simulink model "rotor_simulink"  (R2022a)
settings: Solver=FixedStepAuto  StartTime=0  StopTime=150  FixedStep=time_step  RelTol=1e-3
undefined symbols (not defined in the file or in its folder): blade, gearbox, generator, I_eq, K_opt, lambda_vector, lookup_cP, omega_r, omega_rated, pitch_range, pitch_vector, rho, rotor, wind_speed
settings Model: Creator=Niccolò  LastModifiedBy=Niccolò

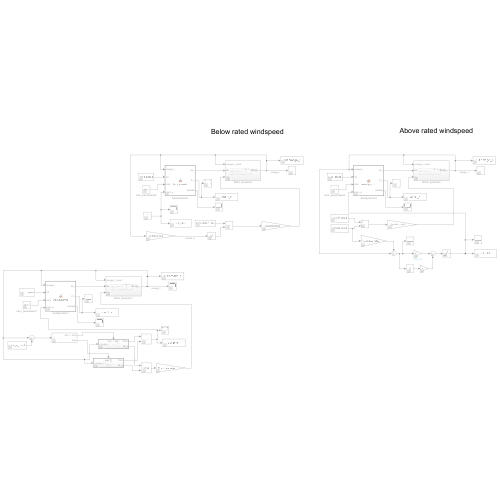
[thumbnail: Simulink's stored preview of the top-level diagram]
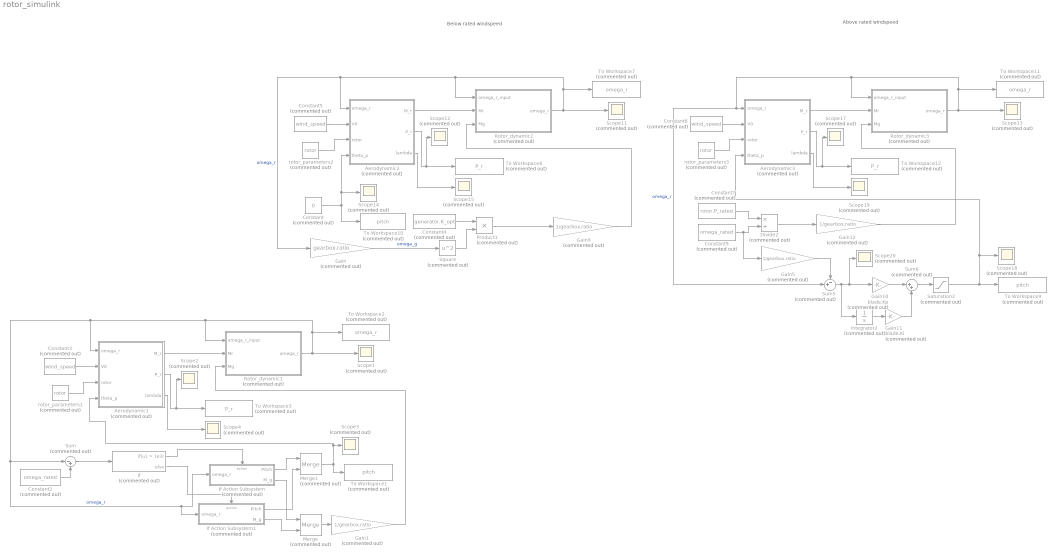
== system rotor_simulink ==
  note: Below rated windspeed
  note: Above rated windspeed
  Aerodynamic1 : MATLAB Function  Commented=on  TreatAsAtomicUnit=on
  Aerodynamic2 : MATLAB Function  Commented=on  TreatAsAtomicUnit=on
  Aerodynamic3 : MATLAB Function  Commented=on  TreatAsAtomicUnit=on
  Constant : Constant  Commented=on  Value=0
  Constant2 : Constant  Commented=on  Value=omega_rated
  Constant3 : Constant  Commented=on  Value=wind_speed
  Constant4 : Constant  Commented=on  Value=generator.K_opt
  Constant5 : Constant  Commented=on  Value=wind_speed
  Constant7 : Constant  Commented=on  Value=rotor.P_rated
  Constant8 : Constant  Commented=on  Value=wind_speed
  Constant9 : Constant  Commented=on  Value=omega_rated
  Divide2 : Product  Commented=on  Inputs=*/
  Gain : Gain  Commented=on  Gain=gearbox.ratio
  Gain{1,5,9,12} (4 alike) : Gain  Commented=on  Gain=1/gearbox.ratio
  Gain10 : Gain  Commented=on  Gain=blade.Kp
  Gain11 : Gain  Commented=on  Gain=blade.Ki
  If : If  Commented=on  IfExpression=u1 > 1e3
  If Action Subsystem : Subsystem  Commented=on  TreatAsAtomicUnit=on
  If Action Subsystem1 : Subsystem  Commented=on  TreatAsAtomicUnit=on
  Integrator2 : Integrator  Commented=on
  Merge : Merge  Commented=on
  Merge1 : Merge  Commented=on
  Product1 : Product  Commented=on
  Rotor_dynamic1 : Subsystem  Commented=on
  Rotor_dynamic2 : Subsystem  Commented=on
  Rotor_dynamic3 : Subsystem  Commented=on
  Saturation2 : Saturate  Commented=on  UpperLimit=30*pi/180  LowerLimit=pitch_range(1)
  Scope{1..4,11..15,17..20} (13 alike) : Scope  Commented=on
  Square : Math  Commented=on  Operator=square
  Sum : Sum  Commented=on  Inputs=|-+
  Sum5 : Sum  Commented=on  Inputs=-+|
  Sum6 : Sum  Commented=on  Inputs=|++
  To Workspace1 : ToWorkspace  Commented=on  VariableName=pitch  SaveFormat=Timeseries  SampleTime=-1
  To Workspace10 : ToWorkspace  Commented=on  VariableName=pitch  SaveFormat=Timeseries  SampleTime=-1
  To Workspace11 : ToWorkspace  Commented=on  VariableName=omega_r  SaveFormat=Timeseries  SampleTime=-1
  To Workspace12 : ToWorkspace  Commented=on  VariableName=P_r  SaveFormat=Timeseries  SampleTime=-1
  To Workspace2 : ToWorkspace  Commented=on  VariableName=omega_r  SaveFormat=Timeseries  SampleTime=-1
  To Workspace3 : ToWorkspace  Commented=on  VariableName=P_r  SaveFormat=Timeseries  SampleTime=-1
  To Workspace7 : ToWorkspace  Commented=on  VariableName=omega_r  SaveFormat=Timeseries  SampleTime=-1
  To Workspace8 : ToWorkspace  Commented=on  VariableName=P_r  SaveFormat=Timeseries  SampleTime=-1
  To Workspace9 : ToWorkspace  Commented=on  VariableName=pitch  SaveFormat=Timeseries  SampleTime=-1
  rotor_parameters1 : Constant  Commented=on  Value=rotor  OutDataTypeStr=Bus: rotor_bus
  rotor_parameters2 : Constant  Commented=on  Value=rotor  OutDataTypeStr=Bus: rotor_bus
  rotor_parameters3 : Constant  Commented=on  Value=rotor  OutDataTypeStr=Bus: rotor_bus
  wires:
  Rotor_dynamic2/1(omega_r) -> Scope11/1, To Workspace7/1, Rotor_dynamic2/1(omega_r_input), Gain/1, Aerodynamic2/1(omega_r)  "omega_r"
  Constant5/1 -> Aerodynamic2/2(V0)
  Aerodynamic2/2(P_r) -> Scope12/1, To Workspace8/1
  Gain9/1 -> Rotor_dynamic2/3(Mg)
  Aerodynamic2/3(lambda) -> Scope15/1
  Aerodynamic2/1(M_r) -> Rotor_dynamic2/2(Mr)
  rotor_parameters2/1 -> Aerodynamic2/3(rotor)
  Saturation2/1 -> To Workspace9/1, Scope18/1, Aerodynamic3/4(theta_p)
  Sum6/1 -> Saturation2/1
  Constant7/1 -> Divide2/1
  Gain5/1 -> Sum5/1
  rotor_parameters3/1 -> Aerodynamic3/3(rotor)
  Integrator2/1 -> Gain11/1
  Aerodynamic3/1(M_r) -> Rotor_dynamic3/2(Mr)
  Aerodynamic3/3(lambda) -> Scope19/1
  Aerodynamic3/2(P_r) -> Scope17/1, To Workspace12/1
  Divide2/1 -> Gain12/1
  Gain10/1 -> Sum6/1
  Gain12/1 -> Rotor_dynamic3/3(Mg)
  Constant8/1 -> Aerodynamic3/2(V0)
  Constant9/1 -> Gain5/1, Divide2/2
  Sum5/1 -> Scope20/1, Gain10/1, Integrator2/1
  Gain11/1 -> Sum6/2
  Rotor_dynamic3/1(omega_r) -> Scope13/1, To Workspace11/1, Rotor_dynamic3/1(omega_r_input), Sum5/2, Aerodynamic3/1(omega_r)  "omega_r"
  Constant/1 -> Aerodynamic2/4(theta_p), Scope14/1, To Workspace10/1
  Constant4/1 -> Product1/1
  Gain/1 -> Square/1  "omega_g"
  Square/1 -> Product1/2
  Product1/1 -> Gain9/1
  Aerodynamic1/2(P_r) -> Scope2/1, To Workspace3/1
  If/1 -> If Action Subsystem/Action
  If/2 -> If Action Subsystem1/Action
  Constant3/1 -> Aerodynamic1/2(V0)
  Aerodynamic1/3(lambda) -> Scope4/1
  rotor_parameters1/1 -> Aerodynamic1/3(rotor)
  Aerodynamic1/1(M_r) -> Rotor_dynamic1/2(Mr)
  Gain1/1 -> Rotor_dynamic1/3(Mg)
  Rotor_dynamic1/1(omega_r) -> Scope1/1, To Workspace2/1, Rotor_dynamic1/1(omega_r_input), Sum/1, If Action Subsystem1/1(omega_r), If Action Subsystem/1(omega_r), Aerodynamic1/1(omega_r)  "omega_r"
  If Action Subsystem/2(M_g) -> Merge/1
  If Action Subsystem1/2(M_g) -> Merge/2
  Merge/1 -> Gain1/1
  Sum/1 -> If/1
  Constant2/1 -> Sum/2
  If Action Subsystem/1(Pitch) -> Merge1/1
  If Action Subsystem1/1(Pitch) -> Merge1/2
  Merge1/1 -> To Workspace1/1, Scope3/1, Aerodynamic1/4(theta_p)

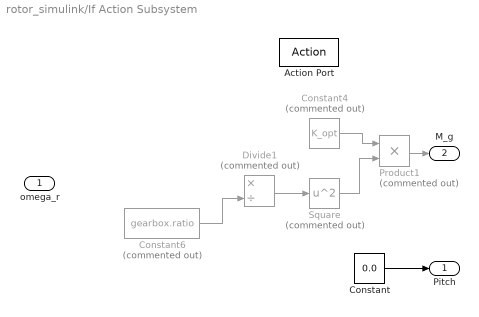
== system rotor_simulink/If Action Subsystem ==
  omega_r : Inport
  Action Port : ActionPort  ActionPortLabel=if(u1 > 1e3)
  Constant : Constant  Value=0.0
  Constant4 : Constant  Commented=on  Value=K_opt
  Constant6 : Constant  Commented=on  Value=gearbox.ratio
  Divide1 : Product  Commented=on  Inputs=*/
  Product1 : Product  Commented=on
  Square : Math  Commented=on  Operator=square
  Pitch : Outport
  M_g : Outport  Port=2
  wires:
  Square/1 -> Product1/2
  Divide1/1 -> Square/1
  Constant4/1 -> Product1/1
  Constant6/1 -> Divide1/2
  Product1/1 -> M_g/1
  Constant/1 -> Pitch/1

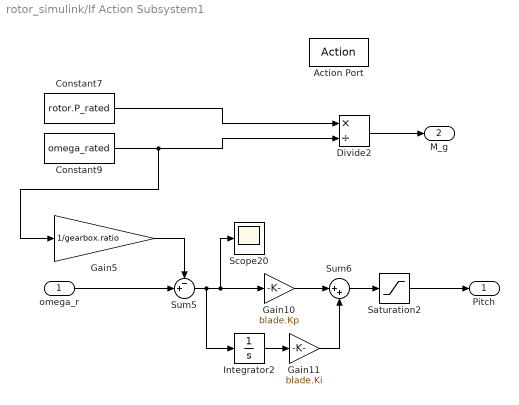
== system rotor_simulink/If Action Subsystem1 ==
  omega_r : Inport
  Action Port : ActionPort  ActionPortLabel=else
  Constant7 : Constant  Value=rotor.P_rated
  Constant9 : Constant  Value=omega_rated
  Divide2 : Product  Inputs=*/
  Gain10 : Gain  Gain=blade.Kp
  Gain11 : Gain  Gain=blade.Ki
  Gain5 : Gain  Gain=1/gearbox.ratio
  Integrator2 : Integrator
  Saturation2 : Saturate  UpperLimit=30*pi/180  LowerLimit=pitch_range(1)
  Scope20 : Scope
  Sum5 : Sum  Inputs=-+|
  Sum6 : Sum  Inputs=|++
  Pitch : Outport
  M_g : Outport  Port=2
  wires:
  Constant7/1 -> Divide2/1
  Divide2/1 -> M_g/1
  Sum6/1 -> Saturation2/1
  Integrator2/1 -> Gain11/1
  Constant9/1 -> Gain5/1, Divide2/2
  Gain11/1 -> Sum6/2
  Sum5/1 -> Scope20/1, Gain10/1, Integrator2/1
  Gain5/1 -> Sum5/1
  Gain10/1 -> Sum6/1
  Saturation2/1 -> Pitch/1
  omega_r/1 -> Sum5/2

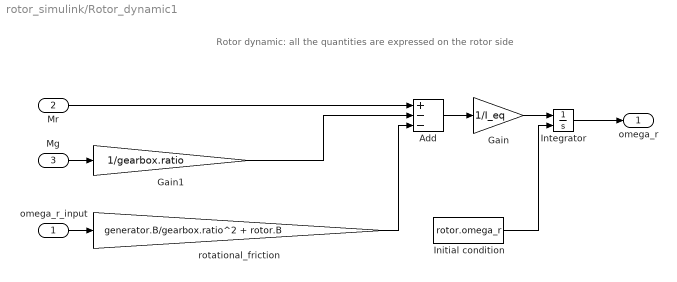
== system rotor_simulink/Rotor_dynamic1 ==
  note: Rotor dynamic: all the quantities are expressed on the rotor side
  omega_r_input : Inport
  Mr : Inport  Port=2
  Mg : Inport  Port=3
  Add : Sum  Inputs=+--
  Gain : Gain  Gain=1/I_eq
  Gain1 : Gain  Gain=1/gearbox.ratio
  Initial condition : Constant  Value=rotor.omega_r
  Integrator : Integrator  InitialConditionSource=external  InitialCondition=omega_r
  rotational_friction : Gain  Gain=generator.B/gearbox.ratio^2 + rotor.B
  omega_r : Outport
  wires:
  Add/1 -> Gain/1
  Gain/1 -> Integrator/1
  Mr/1 -> Add/1
  Initial condition/1 -> Integrator/2
  omega_r_input/1 -> rotational_friction/1
  rotational_friction/1 -> Add/3
  Mg/1 -> Gain1/1
  Gain1/1 -> Add/2
  Integrator/1 -> omega_r/1

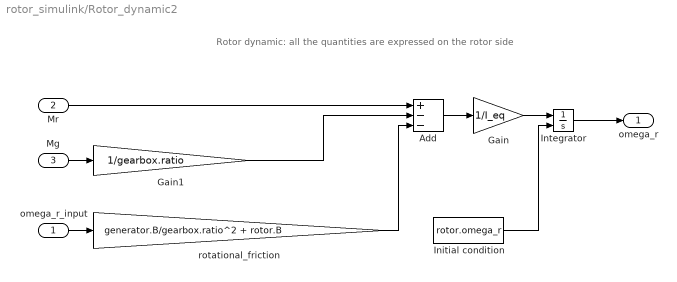
== system rotor_simulink/Rotor_dynamic2 ==
  note: Rotor dynamic: all the quantities are expressed on the rotor side
  omega_r_input : Inport
  Mr : Inport  Port=2
  Mg : Inport  Port=3
  Add : Sum  Inputs=+--
  Gain : Gain  Gain=1/I_eq
  Gain1 : Gain  Gain=1/gearbox.ratio
  Initial condition : Constant  Value=rotor.omega_r
  Integrator : Integrator  InitialConditionSource=external  InitialCondition=omega_r
  rotational_friction : Gain  Gain=generator.B/gearbox.ratio^2 + rotor.B
  omega_r : Outport
  wires:
  Add/1 -> Gain/1
  Gain/1 -> Integrator/1
  Mr/1 -> Add/1
  Initial condition/1 -> Integrator/2
  omega_r_input/1 -> rotational_friction/1
  rotational_friction/1 -> Add/3
  Mg/1 -> Gain1/1
  Gain1/1 -> Add/2
  Integrator/1 -> omega_r/1

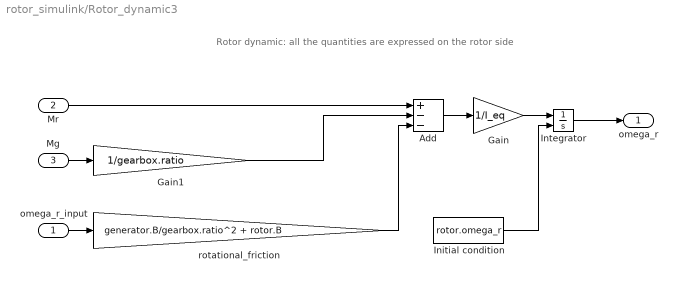
== system rotor_simulink/Rotor_dynamic3 ==
  note: Rotor dynamic: all the quantities are expressed on the rotor side
  omega_r_input : Inport
  Mr : Inport  Port=2
  Mg : Inport  Port=3
  Add : Sum  Inputs=+--
  Gain : Gain  Gain=1/I_eq
  Gain1 : Gain  Gain=1/gearbox.ratio
  Initial condition : Constant  Value=rotor.omega_r
  Integrator : Integrator  InitialConditionSource=external  InitialCondition=omega_r
  rotational_friction : Gain  Gain=generator.B/gearbox.ratio^2 + rotor.B
  omega_r : Outport
  wires:
  Add/1 -> Gain/1
  Gain/1 -> Integrator/1
  Mr/1 -> Add/1
  Initial condition/1 -> Integrator/2
  omega_r_input/1 -> rotational_friction/1
  rotational_friction/1 -> Add/3
  Mg/1 -> Gain1/1
  Gain1/1 -> Add/2
  Integrator/1 -> omega_r/1

== matlab function rotor_simulink/Aerodynamic1 ==
  data: omega_r input; V0 input; M_r output; P_r output; rho parameter; rotor input; theta_p input; lambda_vector parameter; pitch_vector parameter; lookup_cP parameter; lambda output
function [M_r, P_r, lambda] = Aerodynamic(omega_r, V0, rho, rotor, ...
  theta_p, lambda_vector, pitch_vector, lookup_cP) 

R = rotor.R;                  % rotor radius [m]

% retrive the cP from the look-up table
lambda = omega_r*R/V0;                                                
cP = interp2(lambda_vector, pitch_vector, lookup_cP, lambda, theta_p);

P_r = 0.5*rho*V0^3*pi*R^2*cP; % rotor power [W]
M_r = P_r/omega_r;            % rotor torque [Nm]

== matlab function rotor_simulink/Aerodynamic2 ==
  data: omega_r input; V0 input; M_r output; P_r output; rho parameter; rotor input; theta_p input; lambda_vector parameter; pitch_vector parameter; lookup_cP parameter; lambda output
function [M_r, P_r, lambda] = Aerodynamic(omega_r, V0, rho, rotor, ...
  theta_p, lambda_vector, pitch_vector, lookup_cP) 

R = rotor.R;                  % rotor radius [m]

% retrive the cP from the look-up table
lambda = omega_r*R/V0;                                                
cP = interp2(lambda_vector, pitch_vector, lookup_cP, lambda, theta_p);

P_r = 0.5*rho*V0^3*pi*R^2*cP; % rotor power [W]
M_r = P_r/omega_r;            % rotor torque [Nm]

== matlab function rotor_simulink/Aerodynamic3 ==
  data: omega_r input; V0 input; M_r output; P_r output; rho parameter; rotor input; theta_p input; lambda_vector parameter; pitch_vector parameter; lookup_cP parameter; lambda output
function [M_r, P_r, lambda] = Aerodynamic(omega_r, V0, rho, rotor, ...
  theta_p, lambda_vector, pitch_vector, lookup_cP) 

R = rotor.R;                  % rotor radius [m]

% retrive the cP from the look-up table
lambda = omega_r*R/V0;                                                
cP = interp2(lambda_vector, pitch_vector, lookup_cP, lambda, theta_p);

P_r = 0.5*rho*V0^3*pi*R^2*cP; % rotor power [W]
M_r = P_r/omega_r;            % rotor torque [Nm]
